simulink model "gm_Lab2_1"  (R2022a)
settings: Solver=VariableStepAuto  StartTime=0.0  StopTime=10.0  RelTol=1e-3
settings Model: Creator=Dubov  LastModifiedBy=Dubov
settings OptimizationCC: BlockReduction=off  ConditionallyExecuteInputs=off
settings DebuggingCC: InheritedTsInSrcMsg=none

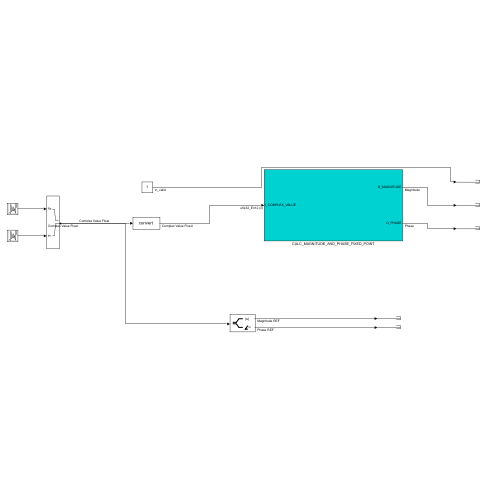
[thumbnail: Simulink's stored preview of the top-level diagram]
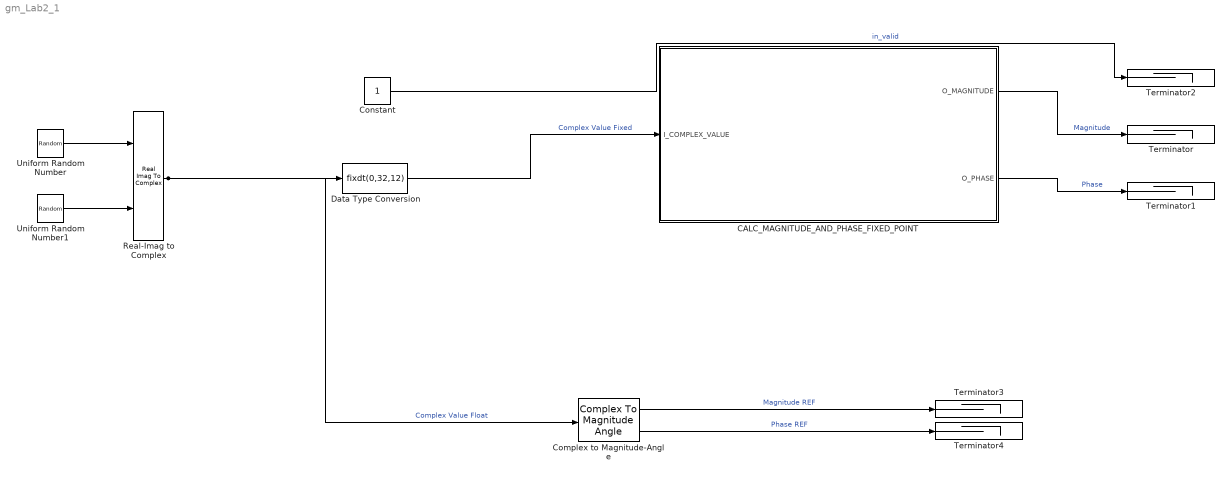
== system gm_Lab2_1 ==
  CALC_MAGNITUDE_AND_PHASE_FIXED_POINT : Subsystem
  Complex to Magnitude-Angle : ComplexToMagnitudeAngle
  Constant : Constant  OutDataTypeStr=boolean
  Data Type Conversion : DataTypeConversion  OutDataTypeStr=fixdt(0,32,12)  RndMeth=Round  SaturateOnIntegerOverflow=off
  Real-Imag to Complex : RealImagToComplex
  Terminator{,1..4} (5 alike) : Terminator
  Uniform Random Number : UniformRandomNumber  Minimum=0  Maximum=2^(20)-1  Seed=20  SampleTime=1
  Uniform Random Number1 : UniformRandomNumber  Minimum=0  Maximum=2^(20)-1  Seed=21  SampleTime=1
  wires:
  Constant/1 -> Terminator2/1  "in_valid"
  CALC_MAGNITUDE_AND_PHASE_FIXED_POINT/2(O_PHASE) -> Terminator1/1  "Phase"
  CALC_MAGNITUDE_AND_PHASE_FIXED_POINT/1(O_MAGNITUDE) -> Terminator/1  "Magnitude"
  Data Type Conversion/1 -> CALC_MAGNITUDE_AND_PHASE_FIXED_POINT/1(I_COMPLEX_VALUE)  "Complex Value Fixed"
  Complex to Magnitude-Angle/2 -> Terminator4/1  "Phase REF"
  Complex to Magnitude-Angle/1 -> Terminator3/1  "Magnitude REF"
  Real-Imag to Complex/1 -> Data Type Conversion/1, Complex to Magnitude-Angle/1  "Complex Value Float"
  Uniform Random Number1/1 -> Real-Imag to Complex/2
  Uniform Random Number/1 -> Real-Imag to Complex/1

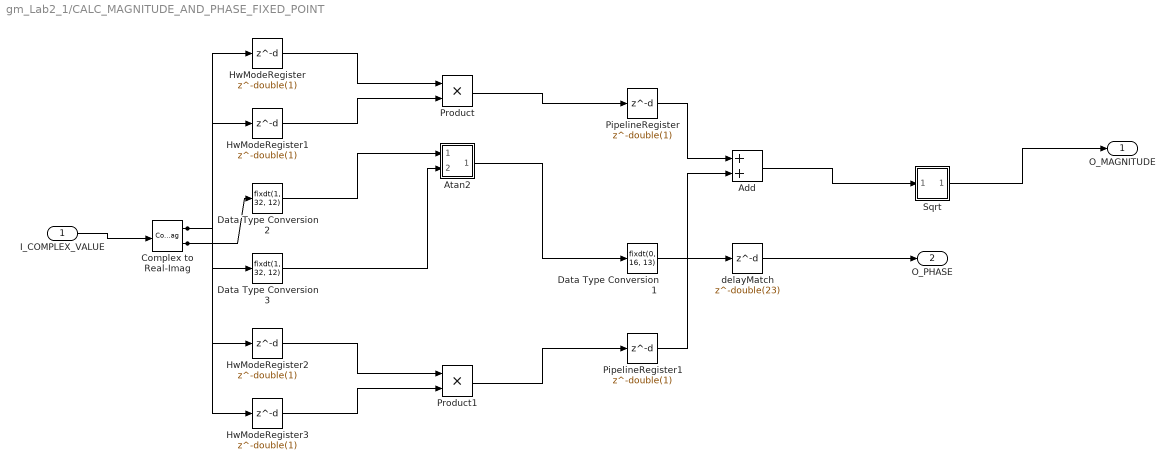
== system gm_Lab2_1/CALC_MAGNITUDE_AND_PHASE_FIXED_POINT ==
  I_COMPLEX_VALUE : Inport  OutDataTypeStr=fixdt(0, 32, 12)  PortDimensions=1  SampleTime=1
      settings: SignalType=complex
  Add : Sum  AccumDataTypeStr=fixdt(0, 65, 24)  OutDataTypeStr=fixdt(0, 65, 24)  SampleTime=1
  Atan2 : Subsystem
  Complex to Real-Imag : ComplexToRealImag  SampleTime=1
  Data Type Conversion1 : DataTypeConversion  OutDataTypeStr=fixdt(0, 16, 13)  RndMeth=Round  SampleTime=1  SaturateOnIntegerOverflow=off
  Data Type Conversion2 : DataTypeConversion  OutDataTypeStr=fixdt(1, 32, 12)  RndMeth=Round  SampleTime=1  SaturateOnIntegerOverflow=off
  Data Type Conversion3 : DataTypeConversion  OutDataTypeStr=fixdt(1, 32, 12)  RndMeth=Round  SampleTime=1  SaturateOnIntegerOverflow=off
  HwModeRegister{,1..3} (4 alike) : Delay  DelayLength=double(1)  InitialCondition=0  SampleTime=1
  PipelineRegister : Delay  DelayLength=double(1)  InitialCondition=0  SampleTime=1
  PipelineRegister1 : Delay  DelayLength=double(1)  InitialCondition=0  SampleTime=1
  Product : Product  Inputs=**  OutDataTypeStr=fixdt(0, 64, 24)  SampleTime=1
  Product1 : Product  Inputs=**  OutDataTypeStr=fixdt(0, 64, 24)  SampleTime=1
  Sqrt : Subsystem
  delayMatch : Delay  DelayLength=double(23)  InitialCondition=0  SampleTime=1
  O_MAGNITUDE : Outport  SampleTime=1
  O_PHASE : Outport  Port=2  SampleTime=1
  wires:
  I_COMPLEX_VALUE/1 -> Complex to Real-Imag/1
  Add/1 -> Sqrt/1(In1)
  Atan2/1(Out1) -> Data Type Conversion1/1
  Complex to Real-Imag/1 -> Data Type Conversion3/1, HwModeRegister/1, HwModeRegister1/1
  Complex to Real-Imag/2 -> Data Type Conversion2/1, HwModeRegister2/1, HwModeRegister3/1
  delayMatch/1 -> O_PHASE/1
  Data Type Conversion2/1 -> Atan2/1(In1)
  Data Type Conversion3/1 -> Atan2/2(In2)
  PipelineRegister/1 -> Add/1
  PipelineRegister1/1 -> Add/2
  Sqrt/1(Out1) -> O_MAGNITUDE/1
  Data Type Conversion1/1 -> delayMatch/1
  Product/1 -> PipelineRegister/1
  HwModeRegister/1 -> Product/1
  HwModeRegister1/1 -> Product/2
  Product1/1 -> PipelineRegister1/1
  HwModeRegister2/1 -> Product1/1
  HwModeRegister3/1 -> Product1/2

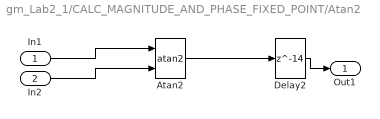
== system gm_Lab2_1/CALC_MAGNITUDE_AND_PHASE_FIXED_POINT/Atan2 ==
  In1 : Inport
  In2 : Inport  Port=2
  Atan2 : Trigonometry  Operator=atan2  ApproximationMethod=CORDIC
  Delay2 : Delay  DelayLength=14
  Out1 : Outport
  wires:
  In1/1 -> Atan2/1
  In2/1 -> Atan2/2
  Atan2/1 -> Delay2/1
  Delay2/1 -> Out1/1

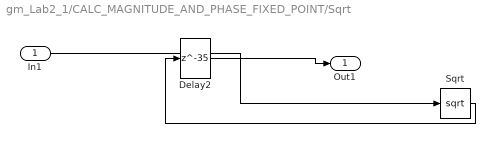
== system gm_Lab2_1/CALC_MAGNITUDE_AND_PHASE_FIXED_POINT/Sqrt ==
  In1 : Inport
  Delay2 : Delay  DelayLength=35
  Sqrt : Sqrt  OutDataTypeStr=Inherit: Inherit via internal rule
  Out1 : Outport
  wires:
  In1/1 -> Sqrt/1
  Sqrt/1 -> Delay2/1
  Delay2/1 -> Out1/1
